simulink model "ValidationModel"  (R2016b)
settings: Solver=ode1  StartTime=0.0  StopTime=Tend  FixedStep=1  RelTol=1e-3
values from neighbouring files (symbols this model uses):
  C1_lookup = theta_lookup(:,4)    [run_validation_model.m]
  Qnom = capacities(i)    [midterm.m]
  R0_lookup = theta_lookup(:,2)    [run_validation_model.m]
  R1_lookup = theta_lookup(:,3)    [run_validation_model.m]
  SOC0 = 1    [midterm.m]
  SOC_curve = Voc_data(:,1)    [run_model.m]    (also in run_validation_model.m)
  SOC_lookup = (0.9:-0.1:0.2)'    [midterm.m]    (also in run_validation_model.m = theta_lookup(:,1))
  Voc_curve = Voc_data(:,2)    [run_model.m]    (also in run_validation_model.m)
libraries: simulink x1
settings Model: Creator=Kramer  LastModifiedBy=Kramer

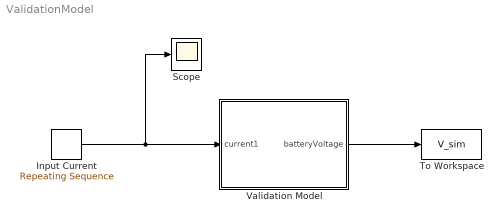
== system ValidationModel ==
  Input Current : simulink/Sources/Repeating Sequence  rep_seq_t=t_data  rep_seq_y=I_data
  Scope : Scope
  To Workspace : ToWorkspace  VariableName=V_sim  SampleTime=-1
  Validation Model : Subsystem
  wires:
  Input Current/1 -> Scope/1, Validation Model/1(current1)
  Validation Model/1(batteryVoltage) -> To Workspace/1

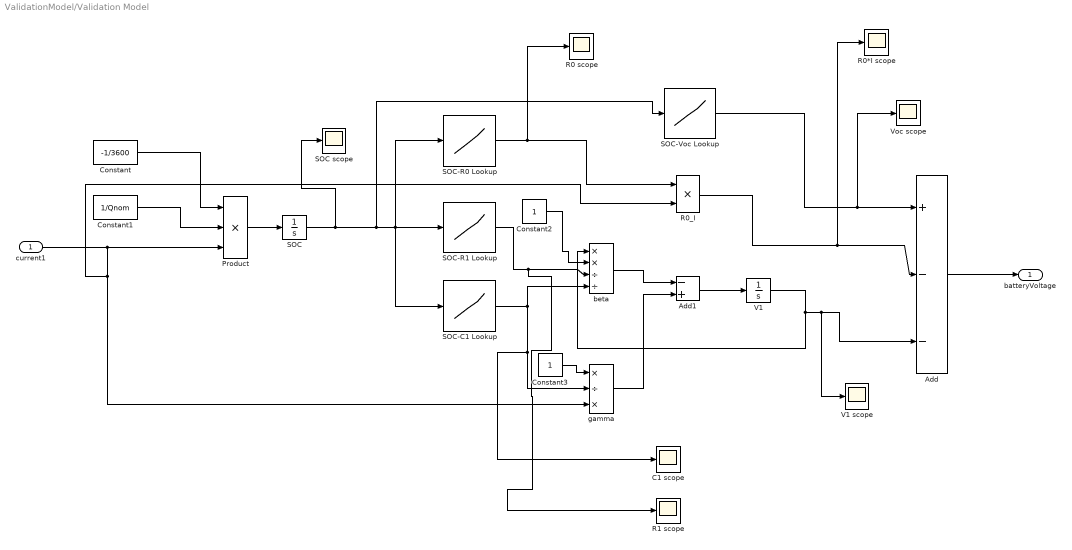
== system ValidationModel/Validation Model ==
  current1 : Inport
  Add : Sum  Inputs=+--
  Add1 : Sum  Inputs=-+
  C1 scope : Scope
  Constant : Constant  Value=-1/3600
  Constant1 : Constant  Value=1/Qnom
  Constant2 : Constant
  Constant3 : Constant
  Product : Product  Inputs=3  RndMeth=Zero
  R0 scope : Scope
  R0*I scope : Scope
  R0_I : Product  RndMeth=Zero
  R1 scope : Scope
  SOC : Integrator  InitialCondition=SOC0
  SOC scope : Scope
  SOC-C1 Lookup : Lookup_n-D  NumberOfTableDimensions=1  BreakpointsForDimension1=SOC_lookup  Table=C1_lookup  InternalRulePriority=Speed  RndMeth=Simplest  InputSameDT=on
  SOC-R0 Lookup : Lookup_n-D  NumberOfTableDimensions=1  BreakpointsForDimension1=SOC_lookup  Table=R0_lookup  InternalRulePriority=Speed  RndMeth=Simplest  InputSameDT=on
  SOC-R1 Lookup : Lookup_n-D  NumberOfTableDimensions=1  BreakpointsForDimension1=SOC_lookup  Table=R1_lookup  InternalRulePriority=Speed  RndMeth=Simplest  InputSameDT=on
  SOC-Voc Lookup : Lookup_n-D  NumberOfTableDimensions=1  BreakpointsForDimension1=SOC_curve  Table=Voc_curve  InternalRulePriority=Speed  RndMeth=Simplest  InputSameDT=on
  V1 : Integrator
  V1 scope : Scope
  Voc scope : Scope
  beta : Product  Inputs=**//
  gamma : Product  Inputs=*/*
  batteryVoltage : Outport
  wires:
  Product/1 -> SOC/1
  Add/1 -> batteryVoltage/1
  Constant1/1 -> Product/2
  V1/1 -> V1 scope/1, Add/3, beta/1
  SOC-Voc Lookup/1 -> Voc scope/1, Add/1
  Constant/1 -> Product/1
  R0_I/1 -> R0*I scope/1, Add/2
  current1/1 -> R0_I/2, gamma/3, Product/3
  SOC/1 -> SOC-Voc Lookup/1, SOC-C1 Lookup/1, SOC-R0 Lookup/1, SOC-R1 Lookup/1, SOC scope/1
  SOC-R0 Lookup/1 -> R0 scope/1, R0_I/1
  Constant2/1 -> beta/2
  SOC-R1 Lookup/1 -> R1 scope/1, beta/3
  SOC-C1 Lookup/1 -> beta/4, C1 scope/1, gamma/2
  Constant3/1 -> gamma/1
  beta/1 -> Add1/1
  gamma/1 -> Add1/2
  Add1/1 -> V1/1
